simulink model "InverterPoster2"  (R2019a)
settings: Solver=VariableStepAuto  StartTime=0.0  StopTime=10.0  RelTol=1e-3
undefined symbols (not defined in the file): J, Ki, Kp, TorqueRef, Ts, Tsc, Vf, Vnom
libraries: fl_lib x21, nesl_utility x11, ee_lib x4, eeTransforms x2, eePwmGeneratorTwoLevel x1
settings Model: Creator=plewi  LastModifiedBy=plewi

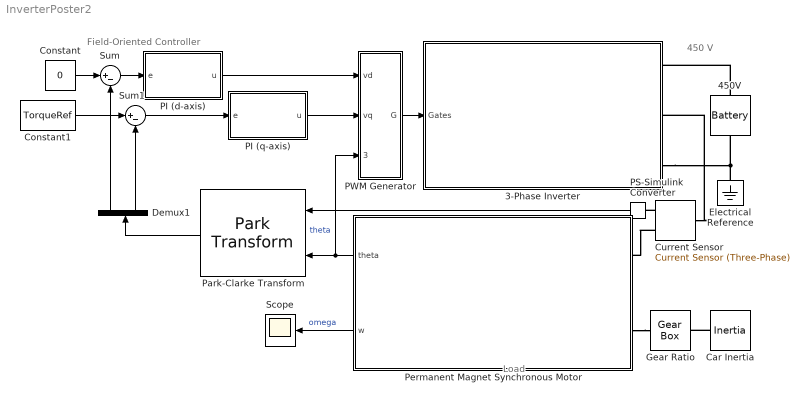
== system InverterPoster2 ==
  note: Field-Oriented Controller
  note: 450 V
  note: Load
  3-Phase Inverter : Subsystem
      mask Display: image('C:\Users\plewi\Documents\University\6-Sixth Year\MUR\MUR-E_Simulation_2019\Images\igbt_inverter.png');
  450V : ee_lib/Sources/Battery  Vnom=12 V  R1=2 Ohm  prm_AH=1  AH=50 hr*A  V1=11.5 V  AH1=25 hr*A  prm_R2=1  R2=2000 Ohm  prm_dyn=1  Rp1=0.005 Ohm  tau1=30 s  Rp2=0.005 Ohm  tau2=30 s  Rp3=0.005 Ohm  tau3=30 s  Rp4=0.005 Ohm  tau4=30 s  Rp5=0.005 Ohm  tau5=30 s  prm_fade=1  N_fade=100  AH_fade=45 hr*A  R1_fade=2.02 Ohm  V1_fade=10.35 V  i_specify=off  i_priority=None  i=0 A  i_nominal_specify=off  i_nominal_unit=A  i_nominal_value=1  v_specify=off  v_priority=None  v=0 V  v_nominal_specify=off  v_nominal_unit=V  v_nominal_value=1  charge_specify=off  charge_priority=High  charge=50 hr*A  charge_nominal_specify=off  charge_nominal_unit=hr*A  charge_nominal_value=1  num_cycles_specify=off  num_cycles_priority=High  num_cycles=0  num_cycles_nominal_specify=off  num_cycles_nominal_unit=1  num_cycles_nominal_value=1  thermal_mass=30000 J/K  Tmeas=298.15 K  Vnom_T2=12 V  R1_T2=2.2 Ohm  V1_T2=11.4 V  R2_T2=2200 Ohm  Rp1_T2=0.005 Ohm  tau1_T2=30 s  Rp2_T2=0.005 Ohm  tau2_T2=30 s  Rp3_T2=0.005 Ohm  tau3_T2=30 s  Rp4_T2=0.005 Ohm  tau4_T2=30 s  Rp5_T2=0.005 Ohm  tau5_T2=30 s  Tmeas2=273.15 K  temperature_specify=off  temperature_priority=High  temperature=298.15 K  temperature_nominal_specify=off  temperature_nominal_unit=K  temperature_nominal_value=1
      settings: SourceProductName=Simscape Electrical
  Car Inertia : fl_lib/Mechanical/Rotational Elements/Inertia  inertia=J kg*m^2  w_specify=off  w_priority=High  w=0 rad/s  w_nominal_specify=off  w_nominal_unit=rad/s  w_nominal_value=1  t_specify=off  t_priority=None  t=0 N*m  t_nominal_specify=off  t_nominal_unit=N*m  t_nominal_value=1
  Constant : Constant  Value=0
  Constant1 : Constant  Value=TorqueRef
  Current Sensor : ee_lib/Sensors & Transducers/Current Sensor (Three-Phase)
      settings: SourceProductName=Simscape Electrical
  Demux1 : Demux  Outputs=2
  Electrical Reference : fl_lib/Electrical/Electrical Elements/Electrical Reference
      settings: SourceProductName=Foundation Library
  Gear Ratio : fl_lib/Mechanical/Mechanisms/Gear Box  ratio=3.27  t_in_specify=off  t_in_priority=None  t_in=0 N*m  t_in_nominal_specify=off  t_in_nominal_unit=N*m  t_in_nominal_value=1  t_out_specify=off  t_out_priority=None  t_out=0 N*m  t_out_nominal_specify=off  t_out_nominal_unit=N*m  t_out_nominal_value=1
  PI (d-axis) : Subsystem
  PI (q-axis) : Subsystem
  PS-Simulink Converter : nesl_utility/PS-Simulink Converter  PhysicalDomain=network_engine_domain  SubClassName=ps_output  LeftPortType=input  RightPortType=output  PseudoPeriodic=off  Frequencies=[]  Unit=1  AffineConversion=off
  PWM Generator : Subsystem
  Park-Clarke Transform : eeTransforms/Park Transform  AxisAlignment=Q-axis  PowerInvariant=on  mask(Park Transform){}
      settings: SourceProductName=Simscape Electrical
      mask Display: image('C:\Users\plewi\Documents\University\6-Sixth Year\MUR\MUR-E_Simulation_2019\Images\ParkClarke.png');
  Permanent Magnet Synchronous Motor : Subsystem
      mask Display: image('C:\Users\plewi\Documents\University\6-Sixth Year\MUR\MUR-E_Simulation_2019\Images\fem_pmsm_schem.png');
  Scope : Scope
  Sum : Sum  Inputs=|+-
  Sum1 : Sum  Inputs=|+-
  wires:
  PWM Generator/1(G) -> 3-Phase Inverter/1(Gates)
  PI (q-axis)/1(u) -> PWM Generator/2(vq)
  PS-Simulink Converter/1 -> Park-Clarke Transform/1
  Permanent Magnet Synchronous Motor/1(theta) -> PWM Generator/3(theta), Park-Clarke Transform/2  "theta"
  Demux1/2 -> Sum1/2
  Demux1/1 -> Sum/2
  Sum1/1 -> PI (q-axis)/1(e)
  Park-Clarke Transform/1 -> Demux1/1
  Constant/1 -> Sum/1
  Constant1/1 -> Sum1/1
  Sum/1 -> PI (d-axis)/1(e)
  PI (d-axis)/1(u) -> PWM Generator/1(vd)
  Permanent Magnet Synchronous Motor/2(w) -> Scope/1  "omega"
  connections:
  Electrical Reference/LConn1 -- 3-Phase Inverter/RConn3 -- 450V/RConn1
  Permanent Magnet Synchronous Motor/LConn2 -- Gear Ratio/LConn1
  Car Inertia/LConn1 -- Gear Ratio/RConn1
  Current Sensor/LConn1 -- 3-Phase Inverter/RConn2
  Current Sensor/RConn2 -- Permanent Magnet Synchronous Motor/LConn1
  Current Sensor/RConn1 -- PS-Simulink Converter/LConn1
  450V/LConn1 -- 3-Phase Inverter/RConn1

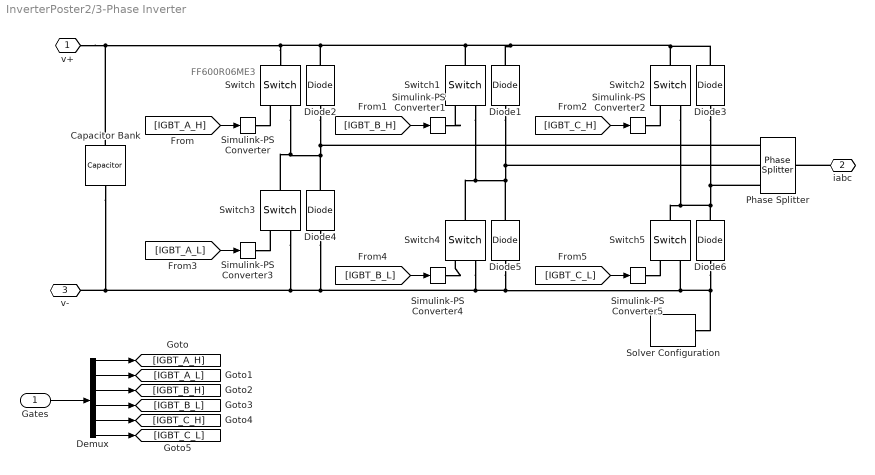
== system InverterPoster2/3-Phase Inverter ==
  note: FF600R06ME3
  Gates : Inport
  Capacitor Bank : fl_lib/Electrical/Electrical Elements/Capacitor  c=320 uF  r=0 Ohm  g=0 1/Ohm  i_specify=off  i_priority=None  i=0 A  i_nominal_specify=off  i_nominal_unit=A  i_nominal_value=1  v_specify=off  v_priority=None  v=0 V  v_nominal_specify=off  v_nominal_unit=V  v_nominal_value=1  vc_specify=on  vc_priority=None  vc=0 V  vc_nominal_specify=off  vc_nominal_unit=V  vc_nominal_value=1
  Demux : Demux  Outputs=6
  Diode{1..6} (6 alike) : fl_lib/Electrical/Electrical Elements/Diode  Vf=diode_Vf V  Ron=diode_Ron Ohm  Goff=diode_Goff 1/Ohm  i_specify=off  i_priority=None  i=0 A  i_nominal_specify=off  i_nominal_unit=A  i_nominal_value=1  v_specify=off  v_priority=None  v=0 V  v_nominal_specify=off  v_nominal_unit=V  v_nominal_value=1
  Phase Splitter : ee_lib/Connectors & References/Phase Splitter
      settings: SourceProductName=Simscape Electrical  SourceProductBaseCode=PS
  Simulink-PS Converter{,1..5} (6 alike) : nesl_utility/Simulink-PS Converter  PhysicalDomain=network_engine_domain  SubClassName=ps_input  LeftPortType=input  RightPortType=output  PseudoPeriodic=off  Frequencies=[]  NoiseDistribution=none  NoiseParameters=[]  Unit=1  AffineConversion=off  FilteringAndDerivatives=provide  SimscapeFilterOrder=1  InputFilterTimeConstant=0.001  UdotUserProvided=0
  Solver Configuration : nesl_utility/Solver Configuration  PhysicalDomain=network_engine_domain  SubClassName=solver  LeftPortType=input  RightPortType=generic  Tones=[]  Harmonics=[]  SimulateNoise=off  Profile=off  UseLocalSampling=off  EnableSwitchedLinearOptims=on  FrequencyDomain=off  UseCCode=off  RelTol=0.001  AbsTol=1e-06  MinStep=1e-09  ToWorkspace=off  RevertToSquareIcSolve=off  NumHomotopyIterations=100  PhasorMode=off  PhasorModeNumHarmonics=1  DoDC=off  ResidualTolerance=1e-09  UseLocalSolver=off  LocalSolverChoice=NE_BACKWARD_EULER_ADVANCER  LocalSolverSampleTime=0.001  DoFixedCost=off  MaxNonlinIter=3  MaxModeIter=2  LinearAlgebra=auto  EquationFormulation=NE_TIME_EF  DelaysMemoryBudget=1024  AutomaticFiltering=on  FilteringTimeConstant=0.001  PartitionStorageMethod=AS_NEEDED  PartitionMemoryBudget=1024  PartitionMethod=ROBUST
  Switch{,1..5} (6 alike) : fl_lib/Electrical/Electrical Elements/Switch  R_closed=Ron Ohm  G_open=Goff 1/Ohm  Threshold=Vf  i_specify=off  i_priority=None  i=0 A  i_nominal_specify=off  i_nominal_unit=A  i_nominal_value=1  v_specify=off  v_priority=None  v=0 V  v_nominal_specify=off  v_nominal_unit=V  v_nominal_value=1
      settings: SourceProductName=Simscape
  v+ : PMIOPort  Tag=PMCPort  Side=Right
  iabc : PMIOPort  Tag=PMCPort  Port=2  Side=Right
  v- : PMIOPort  Tag=PMCPort  Port=3  Side=Right
  wires:
  Demux/6 -> [IGBT_C_L]
  Demux/5 -> [IGBT_C_H]
  Demux/4 -> [IGBT_B_L]
  Demux/3 -> [IGBT_B_H]
  Demux/2 -> [IGBT_A_L]
  Demux/1 -> [IGBT_A_H]
  [IGBT_C_L] -> Simulink-PS Converter5/1
  [IGBT_B_L] -> Simulink-PS Converter4/1
  [IGBT_A_L] -> Simulink-PS Converter3/1
  [IGBT_C_H] -> Simulink-PS Converter2/1
  [IGBT_B_H] -> Simulink-PS Converter1/1
  [IGBT_A_H] -> Simulink-PS Converter/1
  Gates/1 -> Demux/1
  connections:
  Switch5/LConn1 -- Switch2/RConn2 -- Phase Splitter/RConn3 -- Diode3/LConn1 -- Diode6/RConn1
  Diode5/RConn1 -- Phase Splitter/RConn2 -- Diode1/LConn1 -- Switch1/RConn2 -- Switch4/LConn1
  Simulink-PS Converter5/RConn1 -- Switch5/RConn1
  Simulink-PS Converter4/RConn1 -- Switch4/RConn1
  Simulink-PS Converter3/RConn1 -- Switch3/RConn1
  Simulink-PS Converter2/RConn1 -- Switch2/RConn1
  Simulink-PS Converter1/RConn1 -- Switch1/RConn1
  Simulink-PS Converter/RConn1 -- Switch/RConn1
  Switch/LConn1 -- Diode2/RConn1 -- Switch1/LConn1 -- Diode3/RConn1 -- Switch2/LConn1 -- Diode1/RConn1 -- Capacitor Bank/LConn1 -- v+/RConn1
  v-/RConn1 -- Capacitor Bank/RConn1 -- Switch4/RConn2 -- Diode5/LConn1 -- Solver Configuration/RConn1 -- Diode6/LConn1 -- Switch5/RConn2 -- Diode4/LConn1 -- Switch3/RConn2
  Diode2/LConn1 -- Phase Splitter/RConn1 -- Diode4/RConn1 -- Switch3/LConn1 -- Switch/RConn2
  iabc/RConn1 -- Phase Splitter/LConn1

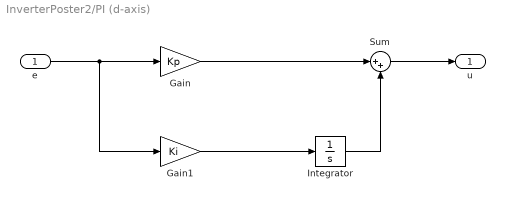
== system InverterPoster2/PI (d-axis) ==
  e : Inport  SampleTime=Ts
  Gain : Gain  Gain=Kp
  Gain1 : Gain  Gain=Ki
  Integrator : Integrator
  Sum : Sum  Inputs=|++
  u : Outport
  wires:
  e/1 -> Gain1/1, Gain/1
  Gain1/1 -> Integrator/1
  Sum/1 -> u/1
  Integrator/1 -> Sum/2
  Gain/1 -> Sum/1

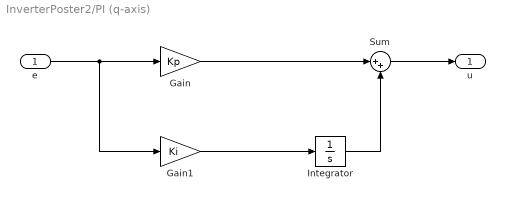
== system InverterPoster2/PI (q-axis) ==
  e : Inport  SampleTime=Ts
  Gain : Gain  Gain=Kp
  Gain1 : Gain  Gain=Ki
  Integrator : Integrator
  Sum : Sum  Inputs=|++
  u : Outport
  wires:
  e/1 -> Gain1/1, Gain/1
  Gain1/1 -> Integrator/1
  Sum/1 -> u/1
  Integrator/1 -> Sum/2
  Gain/1 -> Sum/1

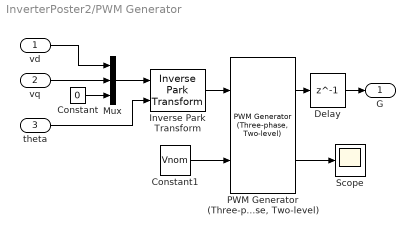
== system InverterPoster2/PWM Generator ==
  vd : Inport
  vq : Inport  Port=2
  theta : Inport  Port=3
  Constant : Constant  Value=0  SampleTime=Tsc
  Constant1 : Constant  Value=Vnom
  Delay : Delay  DelayLength=1
  Inverse Park Transform : eeTransforms/Inverse Park Transform  AxisAlignment=Q-axis  PowerInvariant=off
      settings: SourceProductName=Simscape Electrical
  Mux : Mux  Inputs=3
  "PWM Generator (Three-phase, Two-level)" : eePwmGeneratorTwoLevel/PWM Generator (Three-phase, Two-level)  PWMMode=Continuous PWM (CPWM)  CPWMMode=SVM: space vector modulation  DPWMMode=60 DPWM: 60 degree discontinuous PWM  fsw=fsw  Ts=Ts
      settings: SourceProductName=Simscape Electrical  SourceProductBaseCode=PS
  Scope : Scope
  G : Outport
  wires:
  Inverse Park Transform/1 -> "PWM Generator (Three-phase, Two-level)"/1
  vd/1 -> Mux/1
  theta/1 -> Inverse Park Transform/2
  Constant1/1 -> "PWM Generator (Three-phase, Two-level)"/2
  Mux/1 -> Inverse Park Transform/1
  "PWM Generator (Three-phase, Two-level)"/2 -> Scope/1
  Constant/1 -> Mux/3
  vq/1 -> Mux/2
  "PWM Generator (Three-phase, Two-level)"/1 -> Delay/1
  Delay/1 -> G/1

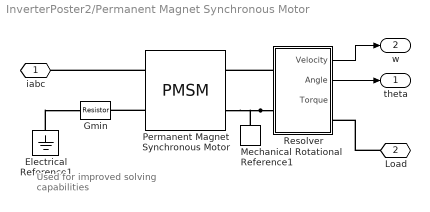
== system InverterPoster2/Permanent Magnet Synchronous Motor ==
  note: Used for improved
      | solving capabilities
  Electrical Reference1 : fl_lib/Electrical/Electrical Elements/Electrical Reference
  Gmin : fl_lib/Electrical/Electrical Elements/Resistor  R=1e9 Ohm  i_specify=off  i_priority=High  i=0 A  i_nominal_specify=off  i_nominal_unit=A  i_nominal_value=1  v_specify=off  v_priority=High  v=0 V  v_nominal_specify=off  v_nominal_unit=V  v_nominal_value=1
  Mechanical Rotational Reference1 : fl_lib/Mechanical/Rotational Elements/Mechanical Rotational Reference
  Permanent Magnet Synchronous Motor : ee_lib/Electromechanical/Permanent Magnet/PMSM  nPolePairs=nPolePairs  pmflux_param=1  pm_flux_linkage=pm_flux_linkage Wb  torque_constant=0.18 N*m/A  back_emf_constant=0.18 V/(rad/s)  stator_param=1  Ld=Ld H  Lq=Lq H  L0=L0 H  Ls=0.0002 H  Lm=0.00002 H  Ms=0.00002 H  Rs=Rs Ohm  zero_sequence=zero_sequence  J=J g*cm^2  lam=0.01 N*m/(rad/s)  axes_param=ee.enum.rotorangle.qaxis  i_d_specify=off  i_d_priority=None  i_d=0 A  i_d_nominal_specify=off  i_d_nominal_unit=A  i_d_nominal_value=1  i_q_specify=off  i_q_priority=None  i_q=0 A  i_q_nominal_specify=off  i_q_nominal_unit=A  i_q_nominal_value=1  torque_specify=off  torque_priority=None  torque=0 N*m  torque_nominal_specify=off  torque_nominal_unit=N*m  torque_nominal_value=1  angular_velocity_specify=on  angular_velocity_priority=High  angular_velocity=0 rpm  angular_velocity_nominal_specify=off  angular_velocity_nominal_unit=rpm  angular_velocity_nominal_value=1  angular_position_specify=on  angular_position_priority=High  angular_position=0 rad  angular_position_nominal_specify=off  angular_position_nominal_unit=deg  angular_position_nominal_value=1
      settings: SourceProductName=Simscape Electrical
  Resolver : Subsystem
  iabc : PMIOPort  Side=Left
  Load : PMIOPort  Port=2  Side=Left
  theta : Outport
  w : Outport  Port=2
  wires:
  Resolver/2(Angle) -> theta/1
  Resolver/1(Velocity) -> w/1
  connections:
  Permanent Magnet Synchronous Motor/LConn1 -- iabc/RConn1
  Resolver/LConn1 -- Permanent Magnet Synchronous Motor/RConn1
  Permanent Magnet Synchronous Motor/LConn2 -- Gmin/RConn1
  Load/RConn1 -- Resolver/RConn1
  Resolver/LConn2 -- Permanent Magnet Synchronous Motor/RConn2 -- Mechanical Rotational Reference1/LConn1
  Electrical Reference1/LConn1 -- Gmin/LConn1

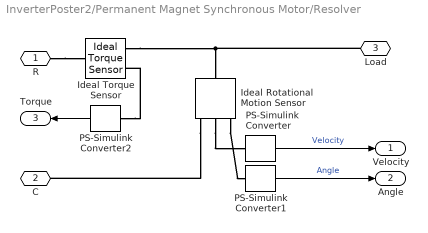
== system InverterPoster2/Permanent Magnet Synchronous Motor/Resolver ==
  Ideal Rotational Motion Sensor : fl_lib/Mechanical/Mechanical Sensors/Ideal Rotational Motion Sensor  offset=0 deg
      settings: SourceProductName=Foundation Library
  Ideal Torque Sensor : fl_lib/Mechanical/Mechanical Sensors/Ideal Torque Sensor
      settings: SourceProductName=Foundation Library
  PS-Simulink Converter : nesl_utility/PS-Simulink Converter  PhysicalDomain=network_engine_domain  SubClassName=ps_output  LeftPortType=input  RightPortType=output  PseudoPeriodic=off  Frequencies=[]  Unit=rad/s  AffineConversion=off
  PS-Simulink Converter1 : nesl_utility/PS-Simulink Converter  PhysicalDomain=network_engine_domain  SubClassName=ps_output  LeftPortType=input  RightPortType=output  PseudoPeriodic=off  Frequencies=[]  Unit=rad  AffineConversion=off
  PS-Simulink Converter2 : nesl_utility/PS-Simulink Converter  PhysicalDomain=network_engine_domain  SubClassName=ps_output  LeftPortType=input  RightPortType=output  PseudoPeriodic=off  Frequencies=[]  Unit=N*m  AffineConversion=off
  R : PMIOPort  Side=Left
  C : PMIOPort  Port=2  Side=Left
  Load : PMIOPort  Port=3  Side=Right
  Velocity : Outport
  Angle : Outport  Port=2
  Torque : Outport  Port=3
  wires:
  PS-Simulink Converter/1 -> Velocity/1  "Velocity"
  PS-Simulink Converter1/1 -> Angle/1  "Angle"
  PS-Simulink Converter2/1 -> Torque/1
  connections:
  Ideal Rotational Motion Sensor/RConn3 -- PS-Simulink Converter1/LConn1
  Ideal Rotational Motion Sensor/RConn2 -- PS-Simulink Converter/LConn1
  Ideal Torque Sensor/RConn1 -- Load/RConn1 -- Ideal Rotational Motion Sensor/LConn1
  Ideal Rotational Motion Sensor/RConn1 -- C/RConn1
  R/RConn1 -- Ideal Torque Sensor/LConn1
  PS-Simulink Converter2/LConn1 -- Ideal Torque Sensor/RConn2
